simulink model "case1"  (R2024b)
settings: Solver=FixedStepAuto  StartTime=0  StopTime=1  FixedStep=1e-7  RelTol=1e-3
values from neighbouring files (symbols this model uses):
  SG_D_1_D = 0.01056    [IEEE9_case_parameters.m]    (also in case1_parameters.m; case2_parameters.m; case3_parameters.m; case4_parameters.m)
  SG_D_1_EnableSaturation = 0    [IEEE9_case_parameters.m]    (also in case1_parameters.m; case2_parameters.m; case3_parameters.m; case4_parameters.m)
  SG_D_1_f0 = 60    [IEEE9_case_parameters.m]    (also in case1_parameters.m; case2_parameters.m; case3_parameters.m; case4_parameters.m)
  SG_D_1_H = 7.5    [IEEE9_case_parameters.m]    (also in case1_parameters.m; case2_parameters.m; case3_parameters.m; case4_parameters.m)
  SG_D_1_K_A = 20    [IEEE9_case_parameters.m]    (also in case1_parameters.m; case2_parameters.m; case3_parameters.m; case4_parameters.m)
  SG_D_1_K_E = 1.000000e+1    (= 10)    [IEEE9_case_parameters.m]    (also in case1_parameters.m; case2_parameters.m; case3_parameters.m; case4_parameters.m)
  SG_D_1_K_F = 2.363    [IEEE9_case_parameters.m]    (also in case1_parameters.m; case2_parameters.m; case3_parameters.m; case4_parameters.m)
  SG_D_1_K_s = 0.5    [IEEE9_case_parameters.m]    (also in case1_parameters.m = 5; case2_parameters.m = 5; case3_parameters.m = 5; case4_parameters.m = 5)
  SG_D_1_R_a = 0.001088    [IEEE9_case_parameters.m]    (also in case1_parameters.m; case2_parameters.m; case3_parameters.m; case4_parameters.m)
  SG_D_1_S_A = 1    [IEEE9_case_parameters.m]    (also in case1_parameters.m; case2_parameters.m; case3_parameters.m; case4_parameters.m)
  SG_D_1_S_B = 0.103    [IEEE9_case_parameters.m]    (also in case1_parameters.m; case2_parameters.m; case3_parameters.m; case4_parameters.m)
  SG_D_1_S_N = 10.659857    [IEEE9_case_parameters.m]    (also in case1_parameters.m; case2_parameters.m; case3_parameters.m; case4_parameters.m)
  SG_D_1_SpeedPara = 200    [IEEE9_case_parameters.m]    (also in case1_parameters.m; case2_parameters.m; case3_parameters.m; case4_parameters.m)
  SG_D_1_T_0 = 0.720173    [IEEE9_case_parameters.m]    (also in case1_parameters.m = 0.755522; case2_parameters.m = 0.808931; case3_parameters.m = 0.869402; case4_parameters.m = 0.729316)
  SG_D_1_T_1 = 0.3    [IEEE9_case_parameters.m]    (also in case1_parameters.m; case2_parameters.m; case3_parameters.m; case4_parameters.m)
  SG_D_1_T_2 = 0.05    [IEEE9_case_parameters.m]    (also in case1_parameters.m; case2_parameters.m; case3_parameters.m; case4_parameters.m)
  SG_D_1_T_3 = 0.02    [IEEE9_case_parameters.m]    (also in case1_parameters.m; case2_parameters.m; case3_parameters.m; case4_parameters.m)
  SG_D_1_T_4 = 0.005    [IEEE9_case_parameters.m]    (also in case1_parameters.m; case2_parameters.m; case3_parameters.m; case4_parameters.m)
  SG_D_1_T_A = 0.02    [IEEE9_case_parameters.m]    (also in case1_parameters.m; case2_parameters.m; case3_parameters.m; case4_parameters.m)
  SG_D_1_T_dd = 8.000000e+0    (= 8)    [IEEE9_case_parameters.m]    (also in case1_parameters.m; case2_parameters.m; case3_parameters.m; case4_parameters.m)
  SG_D_1_T_ddd = 0.04    [IEEE9_case_parameters.m]    (also in case1_parameters.m; case2_parameters.m; case3_parameters.m; case4_parameters.m)
  SG_D_1_T_E = 0.314    [IEEE9_case_parameters.m]    (also in case1_parameters.m; case2_parameters.m; case3_parameters.m; case4_parameters.m)
  SG_D_1_T_F = 0.35    [IEEE9_case_parameters.m]    (also in case1_parameters.m; case2_parameters.m; case3_parameters.m; case4_parameters.m)
  SG_D_1_T_qd = 0.8    [IEEE9_case_parameters.m]    (also in case1_parameters.m; case2_parameters.m; case3_parameters.m; case4_parameters.m)
  SG_D_1_T_qdd = 0.02    [IEEE9_case_parameters.m]    (also in case1_parameters.m; case2_parameters.m; case3_parameters.m; case4_parameters.m)
  SG_D_1_T_speed = 0.1    [IEEE9_case_parameters.m]    (also in case1_parameters.m = 200; case2_parameters.m = 200; case3_parameters.m = 200; case4_parameters.m = 200)
  SG_D_1_T_w = 0.5    [IEEE9_case_parameters.m]    (also in case1_parameters.m; case2_parameters.m; case3_parameters.m; case4_parameters.m)
  SG_D_1_V_ref = 1.990276    [IEEE9_case_parameters.m]    (also in case1_parameters.m = 2.042296; case2_parameters.m = 2.051388; case3_parameters.m = 2.089584; case4_parameters.m = 2.01845)
  SG_D_1_w_ref = 376.991118    [IEEE9_case_parameters.m]    (also in case1_parameters.m; case2_parameters.m; case3_parameters.m; case4_parameters.m)
  SG_D_1_wb = 6.000000e+1    (= 60)    [IEEE9_case_parameters.m]    (also in case1_parameters.m; case2_parameters.m; case3_parameters.m; case4_parameters.m)
  SG_D_1_x_d = 1.9    [IEEE9_case_parameters.m]    (also in case1_parameters.m; case2_parameters.m; case3_parameters.m; case4_parameters.m)
  SG_D_1_x_dd = 0.302    [IEEE9_case_parameters.m]    (also in case1_parameters.m; case2_parameters.m; case3_parameters.m; case4_parameters.m)
  SG_D_1_x_ddd = 0.204    [IEEE9_case_parameters.m]    (also in case1_parameters.m; case2_parameters.m; case3_parameters.m; case4_parameters.m)
  SG_D_1_x_l = 0.05    [IEEE9_case_parameters.m]    (also in case1_parameters.m; case2_parameters.m; case3_parameters.m; case4_parameters.m)
  SG_D_1_x_q = 1.3    [IEEE9_case_parameters.m]    (also in case1_parameters.m; case2_parameters.m; case3_parameters.m; case4_parameters.m)
  SG_D_1_x_qd = 0.5    [IEEE9_case_parameters.m]    (also in case1_parameters.m; case2_parameters.m; case3_parameters.m; case4_parameters.m)
  SG_D_1_x_qdd = 0.3    [IEEE9_case_parameters.m]    (also in case1_parameters.m; case2_parameters.m; case3_parameters.m; case4_parameters.m)
  SG_D_2_D = 0.02    [IEEE9_case_parameters.m]    (also in case1_parameters.m; case2_parameters.m; case3_parameters.m; case4_parameters.m)
  SG_D_2_EnableSaturation = 0    [IEEE9_case_parameters.m]    (also in case1_parameters.m; case2_parameters.m; case3_parameters.m; case4_parameters.m)
  SG_D_2_f0 = 60    [IEEE9_case_parameters.m]    (also in case1_parameters.m; case2_parameters.m; case3_parameters.m; case4_parameters.m)
  SG_D_2_H = 8.000000e+0    (= 8)    [IEEE9_case_parameters.m]    (also in case1_parameters.m; case2_parameters.m; case3_parameters.m; case4_parameters.m)
  SG_D_2_K_A = 20    [IEEE9_case_parameters.m]    (also in case1_parameters.m; case2_parameters.m; case3_parameters.m; case4_parameters.m)
  SG_D_2_K_E = 1.000000e+1    (= 10)    [IEEE9_case_parameters.m]    (also in case1_parameters.m; case2_parameters.m; case3_parameters.m; case4_parameters.m)
  SG_D_2_K_F = 2.363    [IEEE9_case_parameters.m]    (also in case1_parameters.m; case2_parameters.m; case3_parameters.m; case4_parameters.m)
  SG_D_2_K_s = 0.5    [IEEE9_case_parameters.m]    (also in case1_parameters.m = 4; case2_parameters.m = 4; case3_parameters.m = 4; case4_parameters.m = 4)
  SG_D_2_R_a = 0.001088    [IEEE9_case_parameters.m]    (also in case1_parameters.m; case2_parameters.m; case3_parameters.m; case4_parameters.m)
  SG_D_2_S_A = 1    [IEEE9_case_parameters.m]    (also in case1_parameters.m; case2_parameters.m; case3_parameters.m; case4_parameters.m)
  SG_D_2_S_B = 0.103    [IEEE9_case_parameters.m]    (also in case1_parameters.m; case2_parameters.m; case3_parameters.m; case4_parameters.m)
  SG_D_2_S_N = 10.659857    [IEEE9_case_parameters.m]    (also in case1_parameters.m; case2_parameters.m; case3_parameters.m; case4_parameters.m)
  SG_D_2_SpeedPara = 200    [IEEE9_case_parameters.m]    (also in case1_parameters.m; case2_parameters.m; case3_parameters.m; case4_parameters.m)
  SG_D_2_T_0 = 1.632913    [IEEE9_case_parameters.m]    (also in case1_parameters.m = 1.632925; case2_parameters.m = 1.632915; case3_parameters.m = 1.632914; case4_parameters.m = 1.632927)
  SG_D_2_T_1 = 0.2    [IEEE9_case_parameters.m]    (also in case1_parameters.m; case2_parameters.m; case3_parameters.m; case4_parameters.m)
  SG_D_2_T_2 = 0.05    [IEEE9_case_parameters.m]    (also in case1_parameters.m; case2_parameters.m; case3_parameters.m; case4_parameters.m)
  SG_D_2_T_3 = 0.02    [IEEE9_case_parameters.m]    (also in case1_parameters.m; case2_parameters.m; case3_parameters.m; case4_parameters.m)
  SG_D_2_T_4 = 0.005    [IEEE9_case_parameters.m]    (also in case1_parameters.m; case2_parameters.m; case3_parameters.m; case4_parameters.m)
  SG_D_2_T_A = 0.02    [IEEE9_case_parameters.m]    (also in case1_parameters.m; case2_parameters.m; case3_parameters.m; case4_parameters.m)
  SG_D_2_T_dd = 7.9    [IEEE9_case_parameters.m]    (also in case1_parameters.m; case2_parameters.m; case3_parameters.m; case4_parameters.m)
  SG_D_2_T_ddd = 0.04    [IEEE9_case_parameters.m]    (also in case1_parameters.m; case2_parameters.m; case3_parameters.m; case4_parameters.m)
  SG_D_2_T_E = 0.314    [IEEE9_case_parameters.m]    (also in case1_parameters.m; case2_parameters.m; case3_parameters.m; case4_parameters.m)
  SG_D_2_T_F = 0.35    [IEEE9_case_parameters.m]    (also in case1_parameters.m; case2_parameters.m; case3_parameters.m; case4_parameters.m)
  SG_D_2_T_qd = 0.8    [IEEE9_case_parameters.m]    (also in case1_parameters.m; case2_parameters.m; case3_parameters.m; case4_parameters.m)
  SG_D_2_T_qdd = 0.015    [IEEE9_case_parameters.m]    (also in case1_parameters.m; case2_parameters.m; case3_parameters.m; case4_parameters.m)
  SG_D_2_T_speed = 0.1    [IEEE9_case_parameters.m]    (also in case1_parameters.m = 150; case2_parameters.m = 150; case3_parameters.m = 150; case4_parameters.m = 150)
  SG_D_2_T_w = 0.35    [IEEE9_case_parameters.m]    (also in case1_parameters.m; case2_parameters.m; case3_parameters.m; case4_parameters.m)
  SG_D_2_V_ref = 2.58547    [IEEE9_case_parameters.m]    (also in case1_parameters.m = 2.597896; case2_parameters.m = 2.587136; case3_parameters.m = 2.586042; case4_parameters.m = 2.599679)
  SG_D_2_w_ref = 376.991118    [IEEE9_case_parameters.m]    (also in case1_parameters.m; case2_parameters.m; case3_parameters.m; case4_parameters.m)
  SG_D_2_wb = 6.000000e+1    (= 60)    [IEEE9_case_parameters.m]    (also in case1_parameters.m; case2_parameters.m; case3_parameters.m; case4_parameters.m)
  SG_D_2_x_d = 1.8    [IEEE9_case_parameters.m]    (also in case1_parameters.m; case2_parameters.m; case3_parameters.m; case4_parameters.m)
  SG_D_2_x_dd = 0.302    [IEEE9_case_parameters.m]    (also in case1_parameters.m; case2_parameters.m; case3_parameters.m; case4_parameters.m)
  SG_D_2_x_ddd = 0.204    [IEEE9_case_parameters.m]    (also in case1_parameters.m; case2_parameters.m; case3_parameters.m; case4_parameters.m)
  SG_D_2_x_l = 0.05    [IEEE9_case_parameters.m]    (also in case1_parameters.m; case2_parameters.m; case3_parameters.m; case4_parameters.m)
  SG_D_2_x_q = 1.25    [IEEE9_case_parameters.m]    (also in case1_parameters.m; case2_parameters.m; case3_parameters.m; case4_parameters.m)
  SG_D_2_x_qd = 0.5    [IEEE9_case_parameters.m]    (also in case1_parameters.m; case2_parameters.m; case3_parameters.m; case4_parameters.m)
  SG_D_2_x_qdd = 0.3    [IEEE9_case_parameters.m]    (also in case1_parameters.m; case2_parameters.m; case3_parameters.m; case4_parameters.m)
  SG_D_3_D = 0.02    [IEEE9_case_parameters.m]    (also in case1_parameters.m; case2_parameters.m; case3_parameters.m; case4_parameters.m)
  SG_D_3_EnableSaturation = 0    [IEEE9_case_parameters.m]    (also in case1_parameters.m; case2_parameters.m; case3_parameters.m; case4_parameters.m)
  SG_D_3_f0 = 60    [IEEE9_case_parameters.m]    (also in case1_parameters.m; case2_parameters.m; case3_parameters.m; case4_parameters.m)
  SG_D_3_H = 7.7    [IEEE9_case_parameters.m]    (also in case1_parameters.m; case2_parameters.m; case3_parameters.m; case4_parameters.m)
  SG_D_3_K_A = 20    [IEEE9_case_parameters.m]    (also in case1_parameters.m; case2_parameters.m; case3_parameters.m; case4_parameters.m)
  SG_D_3_K_E = 1.000000e+1    (= 10)    [IEEE9_case_parameters.m]    (also in case1_parameters.m; case2_parameters.m; case3_parameters.m; case4_parameters.m)
  SG_D_3_K_F = 2.363    [IEEE9_case_parameters.m]    (also in case1_parameters.m; case2_parameters.m; case3_parameters.m; case4_parameters.m)
  SG_D_3_K_s = 0.2    [IEEE9_case_parameters.m]    (also in case1_parameters.m = 2; case2_parameters.m = 2; case3_parameters.m = 2; case4_parameters.m = 2)
  SG_D_3_R_a = 0.001088    [IEEE9_case_parameters.m]    (also in case1_parameters.m; case2_parameters.m; case3_parameters.m; case4_parameters.m)
  SG_D_3_S_A = 1    [IEEE9_case_parameters.m]    (also in case1_parameters.m; case2_parameters.m; case3_parameters.m; case4_parameters.m)
  SG_D_3_S_B = 0.103    [IEEE9_case_parameters.m]    (also in case1_parameters.m; case2_parameters.m; case3_parameters.m; case4_parameters.m)
  SG_D_3_S_N = 10.659857    [IEEE9_case_parameters.m]    (also in case1_parameters.m; case2_parameters.m; case3_parameters.m; case4_parameters.m)
  SG_D_3_SpeedPara = 200    [IEEE9_case_parameters.m]    (also in case1_parameters.m; case2_parameters.m; case3_parameters.m; case4_parameters.m)
  SG_D_3_T_0 = 0.850788    [IEEE9_case_parameters.m]    (also in case1_parameters.m = 0.850786; case2_parameters.m = 0.850787; case3_parameters.m; case4_parameters.m = 0.850786)
  SG_D_3_T_1 = 0.2    [IEEE9_case_parameters.m]    (also in case1_parameters.m; case2_parameters.m; case3_parameters.m; case4_parameters.m)
  SG_D_3_T_2 = 0.05    [IEEE9_case_parameters.m]    (also in case1_parameters.m; case2_parameters.m; case3_parameters.m; case4_parameters.m)
  SG_D_3_T_3 = 0.02    [IEEE9_case_parameters.m]    (also in case1_parameters.m; case2_parameters.m; case3_parameters.m; case4_parameters.m)
  SG_D_3_T_4 = 0.005    [IEEE9_case_parameters.m]    (also in case1_parameters.m; case2_parameters.m; case3_parameters.m; case4_parameters.m)
  SG_D_3_T_A = 0.02    [IEEE9_case_parameters.m]    (also in case1_parameters.m; case2_parameters.m; case3_parameters.m; case4_parameters.m)
  SG_D_3_T_dd = 8.1    [IEEE9_case_parameters.m]    (also in case1_parameters.m; case2_parameters.m; case3_parameters.m; case4_parameters.m)
  SG_D_3_T_ddd = 0.04    [IEEE9_case_parameters.m]    (also in case1_parameters.m; case2_parameters.m; case3_parameters.m; case4_parameters.m)
  SG_D_3_T_E = 0.314    [IEEE9_case_parameters.m]    (also in case1_parameters.m; case2_parameters.m; case3_parameters.m; case4_parameters.m)
  SG_D_3_T_F = 0.35    [IEEE9_case_parameters.m]    (also in case1_parameters.m; case2_parameters.m; case3_parameters.m; case4_parameters.m)
  SG_D_3_T_qd = 0.8    [IEEE9_case_parameters.m]    (also in case1_parameters.m; case2_parameters.m; case3_parameters.m; case4_parameters.m)
  SG_D_3_T_qdd = 0.015    [IEEE9_case_parameters.m]    (also in case1_parameters.m; case2_parameters.m; case3_parameters.m; case4_parameters.m)
  SG_D_3_T_speed = 0.1    [IEEE9_case_parameters.m]    (also in case1_parameters.m = 180; case2_parameters.m = 180; case3_parameters.m = 180; case4_parameters.m = 180)
  SG_D_3_T_w = 0.4    [IEEE9_case_parameters.m]    (also in case1_parameters.m; case2_parameters.m; case3_parameters.m; case4_parameters.m)
  SG_D_3_V_ref = 1.892727    [IEEE9_case_parameters.m]    (also in case1_parameters.m = 1.906439; case2_parameters.m = 1.895535; case3_parameters.m = 1.892105; case4_parameters.m = 1.906598)
  SG_D_3_w_ref = 376.991118    [IEEE9_case_parameters.m]    (also in case1_parameters.m; case2_parameters.m; case3_parameters.m; case4_parameters.m)
  SG_D_3_wb = 6.000000e+1    (= 60)    [IEEE9_case_parameters.m]    (also in case1_parameters.m; case2_parameters.m; case3_parameters.m; case4_parameters.m)
  SG_D_3_x_d = 1.85    [IEEE9_case_parameters.m]    (also in case1_parameters.m; case2_parameters.m; case3_parameters.m; case4_parameters.m)
  SG_D_3_x_dd = 0.302    [IEEE9_case_parameters.m]    (also in case1_parameters.m; case2_parameters.m; case3_parameters.m; case4_parameters.m)
  SG_D_3_x_ddd = 0.204    [IEEE9_case_parameters.m]    (also in case1_parameters.m; case2_parameters.m; case3_parameters.m; case4_parameters.m)
  SG_D_3_x_l = 0.05    [IEEE9_case_parameters.m]    (also in case1_parameters.m; case2_parameters.m; case3_parameters.m; case4_parameters.m)
  SG_D_3_x_q = 1.2    [IEEE9_case_parameters.m]    (also in case1_parameters.m; case2_parameters.m; case3_parameters.m; case4_parameters.m)
  SG_D_3_x_qd = 0.5    [IEEE9_case_parameters.m]    (also in case1_parameters.m; case2_parameters.m; case3_parameters.m; case4_parameters.m)
  SG_D_3_x_qdd = 0.3    [IEEE9_case_parameters.m]    (also in case1_parameters.m; case2_parameters.m; case3_parameters.m; case4_parameters.m)
(part 11 of 12)

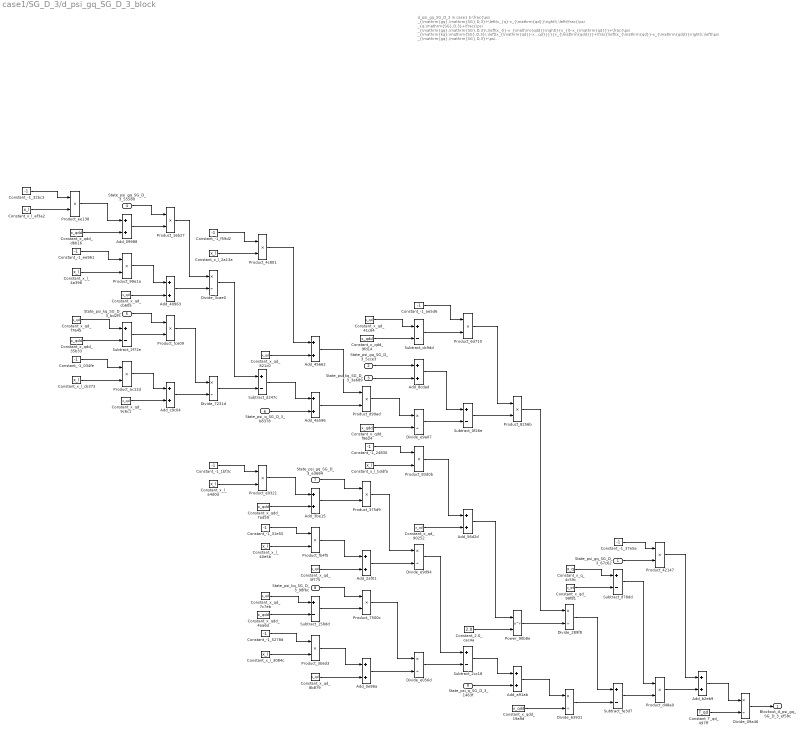
== system case1/SG_D_3/d_psi_gq_SG_D_3_block ==
  note: d_psi_gq_SG_D_3 in case1
      | $-\frac{\psi _{\mathrm{gq},\mathrm{SG},D,3}+\left(x_{q}-x_{\mathrm{qd}}\right)\,\left(\frac{\psi _{q,\mathrm{SG},D,3}+\frac{\psi _{\mathrm{gq},\mathrm{SG},D,3}\,\left(x_{l}-x_{\mathrm{qdd}}\right)}{x_{l}-x_{\mathrm{qd}}}+\frac{\psi _{\mathrm{kq},\mathrm{SG},D,3}\,\left(x_{\mathrm{qd}}-x_{\mathrm{qdd}}\right)}{x_{l}-x_{\mathrm{qd}}}}{x_{\mathrm{qdd}}}+\frac{\left(x_{\mathrm{qd}}-x_{\mathrm{qdd}}\right)\,\left(\psi _{\mathrm{gq},\mathrm{SG},D,3}+\psi _{\mathrm{kq},\mathrm{SG},D,3}+\frac{\left(x_{l}-x_{\mathrm{qd}}\right)\,\left(\psi _{q,\mathrm{SG},D,3}+\frac{\psi _{\mathrm{gq},\mathrm{SG},D,3}\,\left(x_{l}-x_{\mathrm{qdd}}\right)}{x_{l}-x_{\mathrm{qd}}}+\frac{\psi _{\mathrm{kq},\mathrm{SG},D,3}\,\left(x_{\mathrm{qd}}-x_{\mathrm{qdd}}\right)}{x_{l}-x_{\mathrm{qd}}}\right)}{x_{\mathrm{qdd}}}\right)}{{\left(x_{l}-x_{\mathrm{qd}}\right)}^2}\right)}{T_{\mathrm{qd}}}$
      | Automatically generated on 2025-10-31 18:49:40 .
  State_psi_gq_SG_D_3_67c62 : Inport
  State_psi_gq_SG_D_3_5cce3 : Inport  Port=2
  State_psi_kq_SG_D_3_3a689 : Inport  Port=3
  State_psi_gq_SG_D_3_55580 : Inport  Port=4
  State_psi_kq_SG_D_3_bd2f5 : Inport  Port=5
  State_psi_q_SG_D_3_b8378 : Inport  Port=6
  State_psi_gq_SG_D_3_e3684 : Inport  Port=7
  State_psi_kq_SG_D_3_98fbc : Inport  Port=8
  State_psi_q_SG_D_3_1463f : Inport  Port=9
  Add_09988 : Sum
  Add_0e86a : Sum
  Add_2af01 : Sum
  Add_3be15 : Sum
  Add_40963 : Sum
  Add_45662 : Sum
  Add_4a596 : Sum
  Add_56d2d : Sum
  Add_8cdad : Sum
  Add_a91ab : Sum
  Add_b2eb9 : Sum
  Add_c9c04 : Sum
  Constant_-1_034fe : Constant  Value=-1
  Constant_-1_1bf3c : Constant  Value=-1
  Constant_-1_24830 : Constant  Value=-1
  Constant_-1_31e55 : Constant  Value=-1
  Constant_-1_32bc3 : Constant  Value=-1
  Constant_-1_37e5a : Constant  Value=-1
  Constant_-1_5278d : Constant  Value=-1
  Constant_-1_ae5d6 : Constant  Value=-1
  Constant_-1_ee961 : Constant  Value=-1
  Constant_-1_f59d2 : Constant  Value=-1
  Constant_2.0_cac4a : Constant  Value=2.0
  Constant_T_qd_497ff : Constant  Value=T_qd
  Constant_x_l_2a13a : Constant  Value=x_l
  Constant_x_l_3084c : Constant  Value=x_l
  Constant_x_l_40e5b : Constant  Value=x_l
  Constant_x_l_4a396 : Constant  Value=x_l
  Constant_x_l_a4d0d : Constant  Value=x_l
  Constant_x_l_af3a2 : Constant  Value=x_l
  Constant_x_l_b3dfa : Constant  Value=x_l
  Constant_x_l_cb373 : Constant  Value=x_l
  Constant_x_q_4c59c : Constant  Value=x_q
  Constant_x_qd_3f775 : Constant  Value=x_qd
  Constant_x_qd_41c64 : Constant  Value=x_qd
  Constant_x_qd_7c7eb : Constant  Value=x_qd
  Constant_x_qd_821c0 : Constant  Value=x_qd
  Constant_x_qd_8b879 : Constant  Value=x_qd
  Constant_x_qd_90252 : Constant  Value=x_qd
  Constant_x_qd_99f81 : Constant  Value=x_qd
  Constant_x_qd_9c6c1 : Constant  Value=x_qd
  Constant_x_qd_cb605 : Constant  Value=x_qd
  Constant_x_qd_f7645 : Constant  Value=x_qd
  Constant_x_qdd_19a9d : Constant  Value=x_qdd
  Constant_x_qdd_35b33 : Constant  Value=x_qdd
  Constant_x_qdd_4aa6d : Constant  Value=x_qdd
  Constant_x_qdd_7ad59 : Constant  Value=x_qdd
  Constant_x_qdd_9fd14 : Constant  Value=x_qdd
  Constant_x_qdd_dbb16 : Constant  Value=x_qdd
  Constant_x_qdd_f9624 : Constant  Value=x_qdd
  Divide_09a46 : Product  Inputs=*/
  Divide_289f8 : Product  Inputs=*/
  Divide_3cae0 : Product  Inputs=*/
  Divide_63931 : Product  Inputs=*/
  Divide_7231d : Product  Inputs=*/
  Divide_e056d : Product  Inputs=*/
  Divide_e9a07 : Product  Inputs=*/
  Divide_e9d94 : Product  Inputs=*/
  Power_90b8e : Math  Operator=pow
  Product_16b27 : Product
  Product_375d9 : Product
  Product_3b6d3 : Product
  Product_42147 : Product
  Product_4c801 : Product
  Product_6d710 : Product
  Product_7500c : Product
  Product_8256b : Product
  Product_83d0b : Product
  Product_99e1a : Product
  Product_ac12d : Product
  Product_d48a0 : Product
  Product_d99ad : Product
  Product_e0321 : Product
  Product_ee138 : Product
  Product_fb4f5 : Product
  Product_fce09 : Product
  Subtract_0f26e : Sum  Inputs=+-
  Subtract_158dd : Sum  Inputs=+-
  Subtract_2cc18 : Sum  Inputs=+-
  Subtract_2f72e : Sum  Inputs=+-
  Subtract_d247c : Sum  Inputs=+-
  Subtract_d78dd : Sum  Inputs=+-
  Subtract_dc9dd : Sum  Inputs=+-
  Subtract_fe3d7 : Sum  Inputs=+-
  Blockout_d_psi_gq_SG_D_3_ef58c : Outport
  wires:
  Constant_x_l_b3dfa/1 -> Product_83d0b/2
  Constant_x_qd_f7645/1 -> Subtract_2f72e/1
  Add_45662/1 -> Product_d99ad/1
  Constant_-1_32bc3/1 -> Product_ee138/1
  Add_09988/1 -> Product_16b27/2
  Constant_x_qdd_35b33/1 -> Subtract_2f72e/2
  Constant_x_qd_821c0/1 -> Add_45662/2
  Constant_x_l_af3a2/1 -> Product_ee138/2
  Constant_x_l_4a396/1 -> Product_99e1a/2
  Add_0e86a/1 -> Divide_e056d/2
  State_psi_kq_SG_D_3_3a689/1 -> Add_8cdad/2
  Constant_x_qdd_dbb16/1 -> Add_09988/2
  Product_ee138/1 -> Add_09988/1
  Constant_x_qd_8b879/1 -> Add_0e86a/2
  Product_6d710/1 -> Product_8256b/1
  Constant_-1_1bf3c/1 -> Product_e0321/1
  Constant_-1_ee961/1 -> Product_99e1a/1
  Constant_-1_034fe/1 -> Product_ac12d/1
  Constant_x_l_cb373/1 -> Product_ac12d/2
  Constant_-1_ae5d6/1 -> Product_6d710/1
  Constant_-1_37e5a/1 -> Product_42147/1
  State_psi_gq_SG_D_3_55580/1 -> Product_16b27/1
  Product_e0321/1 -> Add_3be15/1
  Product_99e1a/1 -> Add_40963/1
  Product_3b6d3/1 -> Add_0e86a/1
  Constant_x_qd_cb605/1 -> Add_40963/2
  Constant_-1_31e55/1 -> Product_fb4f5/1
  State_psi_kq_SG_D_3_bd2f5/1 -> Product_fce09/1
  Subtract_2f72e/1 -> Product_fce09/2
  Product_ac12d/1 -> Add_c9c04/1
  Add_3be15/1 -> Product_375d9/2
  Add_40963/1 -> Divide_3cae0/2
  Constant_x_qd_9c6c1/1 -> Add_c9c04/2
  Product_16b27/1 -> Divide_3cae0/1
  Constant_T_qd_497ff/1 -> Divide_09a46/2
  Product_fb4f5/1 -> Add_2af01/1
  Product_fce09/1 -> Divide_7231d/1
  Product_7500c/1 -> Divide_e056d/1
  Add_c9c04/1 -> Divide_7231d/2
  Constant_-1_f59d2/1 -> Product_4c801/1
  Constant_x_qdd_f9624/1 -> Divide_e9a07/2
  Constant_x_l_2a13a/1 -> Product_4c801/2
  Divide_3cae0/1 -> Subtract_d247c/1
  Constant_x_qd_99f81/1 -> Subtract_d78dd/2
  Add_2af01/1 -> Divide_e9d94/2
  Divide_7231d/1 -> Subtract_d247c/2
  Constant_x_l_a4d0d/1 -> Product_e0321/2
  Product_4c801/1 -> Add_45662/1
  Constant_-1_24830/1 -> Product_83d0b/1
  Constant_x_l_40e5b/1 -> Product_fb4f5/2
  Subtract_d247c/1 -> Add_4a596/1
  State_psi_q_SG_D_3_b8378/1 -> Add_4a596/2
  Constant_-1_5278d/1 -> Product_3b6d3/1
  Constant_x_qdd_7ad59/1 -> Add_3be15/2
  Constant_x_qd_7c7eb/1 -> Subtract_158dd/1
  Constant_x_qdd_4aa6d/1 -> Subtract_158dd/2
  Constant_x_l_3084c/1 -> Product_3b6d3/2
  Add_4a596/1 -> Product_d99ad/2
  Constant_x_qdd_9fd14/1 -> Subtract_dc9dd/2
  State_psi_gq_SG_D_3_e3684/1 -> Product_375d9/1
  Constant_x_qd_3f775/1 -> Add_2af01/2
  Divide_289f8/1 -> Subtract_fe3d7/1
  State_psi_kq_SG_D_3_98fbc/1 -> Product_7500c/1
  Subtract_158dd/1 -> Product_7500c/2
  Constant_x_qd_41c64/1 -> Subtract_dc9dd/1
  State_psi_gq_SG_D_3_5cce3/1 -> Add_8cdad/1
  Product_d99ad/1 -> Divide_e9a07/1
  Product_375d9/1 -> Divide_e9d94/1
  Subtract_dc9dd/1 -> Product_6d710/2
  Add_8cdad/1 -> Subtract_0f26e/1
  Divide_e9a07/1 -> Subtract_0f26e/2
  Product_83d0b/1 -> Add_56d2d/1
  Constant_x_qd_90252/1 -> Add_56d2d/2
  Divide_e9d94/1 -> Subtract_2cc18/1
  Divide_e056d/1 -> Subtract_2cc18/2
  Subtract_0f26e/1 -> Product_8256b/2
  Add_56d2d/1 -> Power_90b8e/1
  Constant_2.0_cac4a/1 -> Power_90b8e/2
  Subtract_2cc18/1 -> Add_a91ab/1
  State_psi_q_SG_D_3_1463f/1 -> Add_a91ab/2
  Product_8256b/1 -> Divide_289f8/1
  Power_90b8e/1 -> Divide_289f8/2
  Add_a91ab/1 -> Divide_63931/1
  Constant_x_qdd_19a9d/1 -> Divide_63931/2
  Constant_x_q_4c59c/1 -> Subtract_d78dd/1
  Divide_63931/1 -> Subtract_fe3d7/2
  State_psi_gq_SG_D_3_67c62/1 -> Product_42147/2
  Subtract_d78dd/1 -> Product_d48a0/1
  Subtract_fe3d7/1 -> Product_d48a0/2
  Product_42147/1 -> Add_b2eb9/1
  Product_d48a0/1 -> Add_b2eb9/2
  Add_b2eb9/1 -> Divide_09a46/1
  Divide_09a46/1 -> Blockout_d_psi_gq_SG_D_3_ef58c/1

== system case1/SG_D_3/d_psi_kq_SG_D_3_block ==
  note: d_psi_kq_SG_D_3 in case1
      | $-\frac{\psi _{\mathrm{gq},\mathrm{SG},D,3}+\psi _{\mathrm{kq},\mathrm{SG},D,3}+\frac{\left(x_{l}-x_{\mathrm{qd}}\right)\,\left(\psi _{q,\mathrm{SG},D,3}+\frac{\psi _{\mathrm{gq},\mathrm{SG},D,3}\,\left(x_{l}-x_{\mathrm{qdd}}\right)}{x_{l}-x_{\mathrm{qd}}}+\frac{\psi _{\mathrm{kq},\mathrm{SG},D,3}\,\left(x_{\mathrm{qd}}-x_{\mathrm{qdd}}\right)}{x_{l}-x_{\mathrm{qd}}}\right)}{x_{\mathrm{qdd}}}}{T_{\mathrm{qdd}}}$
      | Automatically generated on 2025-10-31 18:49:43 .
  State_psi_gq_SG_D_3_d2333 : Inport
  State_psi_kq_SG_D_3_6b251 : Inport  Port=2
  State_psi_gq_SG_D_3_852d7 : Inport  Port=3
  State_psi_kq_SG_D_3_8c307 : Inport  Port=4
  State_psi_q_SG_D_3_3b888 : Inport  Port=5
  Add_4bba0 : Sum
  Add_58b4c : Sum
  Add_931fd : Sum
  Add_c4f83 : Sum
  Add_e4726 : Sum
  Add_ee729 : Sum
  Constant_-1_2f69e : Constant  Value=-1
  Constant_-1_44d35 : Constant  Value=-1
  Constant_-1_7b10b : Constant  Value=-1
  Constant_-1_a5749 : Constant  Value=-1
  Constant_-1_c2ef4 : Constant  Value=-1
  Constant_T_qdd_8b7ea : Constant  Value=T_qdd
  Constant_x_l_87358 : Constant  Value=x_l
  Constant_x_l_99aa2 : Constant  Value=x_l
  Constant_x_l_d013b : Constant  Value=x_l
  Constant_x_l_fda08 : Constant  Value=x_l
  Constant_x_qd_5ce38 : Constant  Value=x_qd
  Constant_x_qd_80038 : Constant  Value=x_qd
  Constant_x_qd_86b0b : Constant  Value=x_qd
  Constant_x_qd_a3cb9 : Constant  Value=x_qd
  Constant_x_qdd_1b57a : Constant  Value=x_qdd
  Constant_x_qdd_1e56c : Constant  Value=x_qdd
  Constant_x_qdd_b3d62 : Constant  Value=x_qdd
  Divide_14e25 : Product  Inputs=*/
  Divide_2ff9d : Product  Inputs=*/
  Divide_9901f : Product  Inputs=*/
  Divide_bd8a6 : Product  Inputs=*/
  Product_15a3d : Product
  Product_300be : Product
  Product_62232 : Product
  Product_7e491 : Product
  Product_9ff31 : Product
  Product_a4b5c : Product
  Product_b2cfb : Product
  Product_bbfa0 : Product
  Subtract_3fc00 : Sum  Inputs=+-
  Subtract_66370 : Sum  Inputs=+-
  Subtract_b15d7 : Sum  Inputs=+-
  Blockout_d_psi_kq_SG_D_3_28baf : Outport
  wires:
  State_psi_q_SG_D_3_3b888/1 -> Add_4bba0/2
  Constant_-1_c2ef4/1 -> Product_bbfa0/1
  Constant_-1_a5749/1 -> Product_a4b5c/1
  Constant_-1_2f69e/1 -> Product_62232/1
  Constant_x_l_99aa2/1 -> Product_bbfa0/2
  Constant_x_qdd_b3d62/1 -> Add_c4f83/2
  Product_9ff31/1 -> Add_58b4c/1
  Constant_x_l_87358/1 -> Product_a4b5c/2
  Constant_x_qd_86b0b/1 -> Subtract_66370/1
  Product_a4b5c/1 -> Add_c4f83/1
  Constant_x_l_d013b/1 -> Product_15a3d/2
  Constant_x_qdd_1e56c/1 -> Subtract_66370/2
  Constant_-1_44d35/1 -> Product_9ff31/1
  Constant_x_l_fda08/1 -> Product_9ff31/2
  State_psi_gq_SG_D_3_852d7/1 -> Product_b2cfb/1
  Add_c4f83/1 -> Product_b2cfb/2
  Add_4bba0/1 -> Product_7e491/2
  Product_bbfa0/1 -> Add_e4726/1
  Constant_x_qd_80038/1 -> Add_e4726/2
  State_psi_kq_SG_D_3_8c307/1 -> Product_300be/1
  Subtract_66370/1 -> Product_300be/2
  Add_e4726/1 -> Divide_14e25/2
  Constant_x_qd_5ce38/1 -> Add_58b4c/2
  Product_b2cfb/1 -> Divide_14e25/1
  Product_300be/1 -> Divide_bd8a6/1
  Add_58b4c/1 -> Divide_bd8a6/2
  Constant_-1_7b10b/1 -> Product_15a3d/1
  Divide_14e25/1 -> Subtract_3fc00/1
  Add_931fd/1 -> Divide_2ff9d/1
  Divide_bd8a6/1 -> Subtract_3fc00/2
  Divide_2ff9d/1 -> Blockout_d_psi_kq_SG_D_3_28baf/1
  Product_15a3d/1 -> Add_ee729/1
  Constant_x_qd_a3cb9/1 -> Add_ee729/2
  Subtract_3fc00/1 -> Add_4bba0/1
  State_psi_gq_SG_D_3_d2333/1 -> Product_62232/2
  Add_ee729/1 -> Product_7e491/1
  Constant_T_qdd_8b7ea/1 -> Divide_2ff9d/2
  Product_62232/1 -> Subtract_b15d7/1
  State_psi_kq_SG_D_3_6b251/1 -> Subtract_b15d7/2
  Product_7e491/1 -> Divide_9901f/1
  Constant_x_qdd_1b57a/1 -> Divide_9901f/2
  Subtract_b15d7/1 -> Add_931fd/1
  Divide_9901f/1 -> Add_931fd/2

== system case1/SG_D_3/d_psi_q_SG_D_3_block ==
  note: d_psi_q_SG_D_3 in case1
      | $2\,\pi \,f_{0}\,\left(v_{d,\mathrm{SG},D,3}\,\cos\left(\theta _{\mathrm{SG},D,3}\right)+v_{q,\mathrm{SG},D,3}\,\sin\left(\theta _{\mathrm{SG},D,3}\right)-\frac{R_{a}\,\left(\psi _{q,\mathrm{SG},D,3}+\frac{\psi _{\mathrm{gq},\mathrm{SG},D,3}\,\left(x_{l}-x_{\mathrm{qdd}}\right)}{x_{l}-x_{\mathrm{qd}}}+\frac{\psi _{\mathrm{kq},\mathrm{SG},D,3}\,\left(x_{\mathrm{qd}}-x_{\mathrm{qdd}}\right)}{x_{l}-x_{\mathrm{qd}}}\right)}{x_{\mathrm{qdd}}}-\frac{\psi _{d,\mathrm{SG},D,3}\,w_{\mathrm{SG},D,3}}{2\,f_{0}\,\pi }\right)$
      | Automatically generated on 2025-10-31 18:49:26 .
  State_psi_gq_SG_D_3_b4a4d : Inport
  State_psi_kq_SG_D_3_e7fae : Inport  Port=2
  State_psi_q_SG_D_3_1c339 : Inport  Port=3
  Input_v_d_SG_D_3_3c95f : Inport  Port=4
  State_theta_SG_D_3_b412e : Inport  Port=5
  Input_v_q_SG_D_3_30458 : Inport  Port=6
  State_theta_SG_D_3_6cd7f : Inport  Port=7
  State_psi_d_SG_D_3_39242 : Inport  Port=8
  State_w_SG_D_3_33157 : Inport  Port=9
  Add_0a28a : Sum
  Add_1fb4a : Sum
  Add_8a80d : Sum
  Add_8f6d7 : Sum
  Add_b61a3 : Sum
  Constant_-1_09831 : Constant  Value=-1
  Constant_-1_40f79 : Constant  Value=-1
  Constant_-1_7d572 : Constant  Value=-1
  Constant_-2.0_37784 : Constant  Value=-2.0
  Constant_2.0_33906 : Constant  Value=2.0
  Constant_R_a_c673f : Constant  Value=R_a
  Constant_f0_3483c : Constant  Value=f0
  Constant_f0_e42c1 : Constant  Value=f0
  Constant_pi_25a8b : Constant  Value=pi
  Constant_pi_8fec9 : Constant  Value=pi
  Constant_x_l_6b2fb : Constant  Value=x_l
  Constant_x_l_86c92 : Constant  Value=x_l
  Constant_x_l_e01b2 : Constant  Value=x_l
  Constant_x_qd_01ec4 : Constant  Value=x_qd
  Constant_x_qd_6f222 : Constant  Value=x_qd
  Constant_x_qd_86970 : Constant  Value=x_qd
  Constant_x_qdd_033a0 : Constant  Value=x_qdd
  Constant_x_qdd_43d51 : Constant  Value=x_qdd
  Constant_x_qdd_c6aeb : Constant  Value=x_qdd
  Divide_03a1d : Product  Inputs=*/
  Divide_1b431 : Product  Inputs=*/
  Divide_876d5 : Product  Inputs=*/
  Divide_96f7b : Product  Inputs=*/
  MathFunc_cos_99fba : Trigonometry  Operator=cos
  MathFunc_sin_92f53 : Trigonometry
  Product_1a6b3 : Product
  Product_1b548 : Product
  Product_3a97b : Product
  Product_43277 : Product
  Product_692ab : Product
  Product_6ba89 : Product
  Product_91de5 : Product
  Product_984a4 : Product
  Product_a08c0 : Product
  Product_b7b95 : Product
  Product_b9ec1 : Product
  Product_e2263 : Product
  Product_ef29d : Product
  Product_f3098 : Product
  Subtract_16a69 : Sum  Inputs=+-
  Subtract_19dca : Sum  Inputs=+-
  Subtract_55713 : Sum  Inputs=+-
  Subtract_a9ca8 : Sum  Inputs=+-
  Blockout_d_psi_q_SG_D_3_3a763 : Outport
  wires:
  Constant_x_qd_86970/1 -> Subtract_a9ca8/1
  Constant_pi_8fec9/1 -> Product_f3098/2
  Product_1a6b3/1 -> Divide_96f7b/1
  Constant_x_l_e01b2/1 -> Product_43277/2
  Constant_f0_e42c1/1 -> Product_3a97b/2
  State_w_SG_D_3_33157/1 -> Product_e2263/2
  Constant_-1_7d572/1 -> Product_984a4/1
  Constant_x_qdd_033a0/1 -> Add_0a28a/2
  Input_v_d_SG_D_3_3c95f/1 -> Product_6ba89/1
  Constant_x_qdd_c6aeb/1 -> Subtract_a9ca8/2
  Constant_x_l_86c92/1 -> Product_984a4/2
  Divide_1b431/1 -> Add_8f6d7/2
  Product_984a4/1 -> Add_0a28a/1
  Constant_2.0_33906/1 -> Product_f3098/1
  Add_8a80d/1 -> Product_1a6b3/2
  Constant_-1_40f79/1 -> Product_43277/1
  Constant_x_qd_01ec4/1 -> Add_1fb4a/2
  Constant_-1_09831/1 -> Product_1b548/1
  Subtract_16a69/1 -> Subtract_55713/1
  Constant_x_l_6b2fb/1 -> Product_1b548/2
  Subtract_55713/1 -> Add_8f6d7/1
  Constant_f0_3483c/1 -> Product_b9ec1/2
  State_theta_SG_D_3_6cd7f/1 -> MathFunc_sin_92f53/1
  Constant_x_qd_6f222/1 -> Add_b61a3/2
  State_psi_gq_SG_D_3_b4a4d/1 -> Product_a08c0/1
  Add_0a28a/1 -> Product_a08c0/2
  Product_f3098/1 -> Product_b9ec1/1
  Product_43277/1 -> Add_b61a3/1
  State_psi_kq_SG_D_3_e7fae/1 -> Product_ef29d/1
  Subtract_a9ca8/1 -> Product_ef29d/2
  Product_1b548/1 -> Add_1fb4a/1
  MathFunc_sin_92f53/1 -> Product_692ab/2
  Product_a08c0/1 -> Divide_876d5/1
  Product_b9ec1/1 -> Divide_1b431/2
  Add_b61a3/1 -> Divide_876d5/2
  Product_ef29d/1 -> Divide_03a1d/1
  Add_1fb4a/1 -> Divide_03a1d/2
  Input_v_q_SG_D_3_30458/1 -> Product_692ab/1
  Divide_876d5/1 -> Subtract_19dca/1
  Subtract_19dca/1 -> Add_8a80d/1
  Divide_03a1d/1 -> Subtract_19dca/2
  Divide_96f7b/1 -> Subtract_16a69/1
  State_psi_q_SG_D_3_1c339/1 -> Add_8a80d/2
  Product_692ab/1 -> Subtract_55713/2
  Constant_R_a_c673f/1 -> Product_1a6b3/1
  State_theta_SG_D_3_b412e/1 -> MathFunc_cos_99fba/1
  Constant_x_qdd_43d51/1 -> Divide_96f7b/2
  MathFunc_cos_99fba/1 -> Product_6ba89/2
  Constant_-2.0_37784/1 -> Product_91de5/1
  Product_6ba89/1 -> Subtract_16a69/2
  State_psi_d_SG_D_3_39242/1 -> Product_e2263/1
  Constant_pi_25a8b/1 -> Product_91de5/2
  Product_e2263/1 -> Divide_1b431/1
  Product_91de5/1 -> Product_3a97b/1
  Product_3a97b/1 -> Product_b7b95/1
  Add_8f6d7/1 -> Product_b7b95/2
  Product_b7b95/1 -> Blockout_d_psi_q_SG_D_3_3a763/1

== system case1/SG_D_3/d_theta_SG_D_3_block ==
  note: d_theta_SG_D_3 in case1
      | $w_{\mathrm{SG},D,3}-2\,\pi \,f_{0}$
      | Automatically generated on 2025-10-31 18:49:51 .
  State_w_SG_D_3_f4ecf : Inport
  Add_96a9b : Sum
  Constant_-2.0_896de : Constant  Value=-2.0
  Constant_f0_472a7 : Constant  Value=f0
  Constant_pi_f7a3a : Constant  Value=pi
  Product_17f2b : Product
  Product_afb3b : Product
  Blockout_d_theta_SG_D_3_d61c2 : Outport
  wires:
  Constant_-2.0_896de/1 -> Product_17f2b/1
  Constant_pi_f7a3a/1 -> Product_17f2b/2
  State_w_SG_D_3_f4ecf/1 -> Add_96a9b/2
  Product_17f2b/1 -> Product_afb3b/1
  Constant_f0_472a7/1 -> Product_afb3b/2
  Product_afb3b/1 -> Add_96a9b/1
  Add_96a9b/1 -> Blockout_d_theta_SG_D_3_d61c2/1

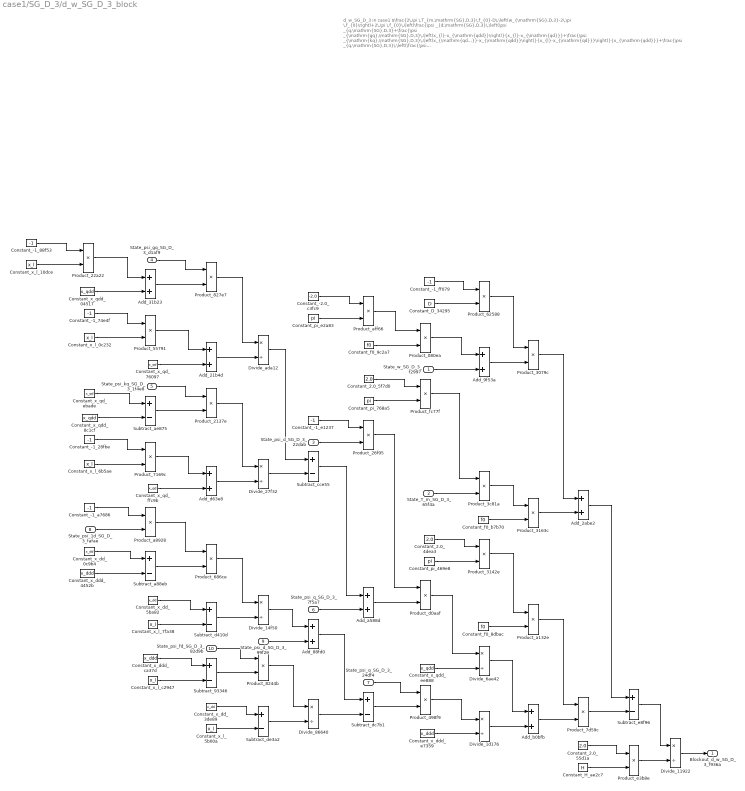
== system case1/SG_D_3/d_w_SG_D_3_block ==
  note: d_w_SG_D_3 in case1
      | $\frac{2\,\pi \,T_{m,\mathrm{SG},D,3}\,f_{0}-D\,\left(w_{\mathrm{SG},D,3}-2\,\pi \,f_{0}\right)+2\,\pi \,f_{0}\,\left(\frac{\psi _{d,\mathrm{SG},D,3}\,\left(\psi _{q,\mathrm{SG},D,3}+\frac{\psi _{\mathrm{gq},\mathrm{SG},D,3}\,\left(x_{l}-x_{\mathrm{qdd}}\right)}{x_{l}-x_{\mathrm{qd}}}+\frac{\psi _{\mathrm{kq},\mathrm{SG},D,3}\,\left(x_{\mathrm{qd}}-x_{\mathrm{qdd}}\right)}{x_{l}-x_{\mathrm{qd}}}\right)}{x_{\mathrm{qdd}}}+\frac{\psi _{q,\mathrm{SG},D,3}\,\left(\frac{\psi _{\mathrm{1d},\mathrm{SG},D,3}\,\left(x_{\mathrm{dd}}-x_{\mathrm{ddd}}\right)}{x_{\mathrm{dd}}-x_{l}}-\psi _{d,\mathrm{SG},D,3}+\frac{\psi _{\mathrm{fd},\mathrm{SG},D,3}\,\left(x_{\mathrm{ddd}}-x_{l}\right)}{x_{\mathrm{dd}}-x_{l}}\right)}{x_{\mathrm{ddd}}}\right)}{2\,H}$
      | Automatically generated on 2025-10-31 18:49:50 .
  State_w_SG_D_3_f2997 : Inport
  State_T_m_SG_D_3_65f4a : Inport  Port=2
  State_psi_d_SG_D_3_22dab : Inport  Port=3
  State_psi_gq_SG_D_3_d1af9 : Inport  Port=4
  State_psi_kq_SG_D_3_1f4e8 : Inport  Port=5
  State_psi_q_SG_D_3_7f5a7 : Inport  Port=6
  State_psi_q_SG_D_3_24df4 : Inport  Port=7
  State_psi_1d_SG_D_3_fafae : Inport  Port=8
  State_psi_d_SG_D_3_99f2e : Inport  Port=9
  State_psi_fd_SG_D_3_82d9b : Inport  Port=10
  Add_21b4d : Sum
  Add_2abe2 : Sum
  Add_31b23 : Sum
  Add_88fd0 : Sum
  Add_9f53a : Sum
  Add_a588d : Sum
  Add_b0bfb : Sum
  Add_d63e8 : Sum
  Constant_-1_28fbe : Constant  Value=-1
  Constant_-1_74e4f : Constant  Value=-1
  Constant_-1_88f53 : Constant  Value=-1
  Constant_-1_a7686 : Constant  Value=-1
  Constant_-1_e1237 : Constant  Value=-1
  Constant_-1_ff079 : Constant  Value=-1
  Constant_-2.0_c3fc9 : Constant  Value=-2.0
  Constant_2.0_4dea3 : Constant  Value=2.0
  Constant_2.0_55d1a : Constant  Value=2.0
  Constant_2.0_5f7d0 : Constant  Value=2.0
  Constant_D_34295 : Constant  Value=D
  Constant_H_ae2c7 : Constant  Value=H
  Constant_f0_8dbac : Constant  Value=f0
  Constant_f0_9c2a7 : Constant  Value=f0
  Constant_f0_b7b70 : Constant  Value=f0
  Constant_pi_469e8 : Constant  Value=pi
  Constant_pi_768a5 : Constant  Value=pi
  Constant_pi_e2a83 : Constant  Value=pi
  Constant_x_dd_0c9b4 : Constant  Value=x_dd
  Constant_x_dd_3de89 : Constant  Value=x_dd
  Constant_x_dd_5ba82 : Constant  Value=x_dd
  Constant_x_ddd_4452b : Constant  Value=x_ddd
  Constant_x_ddd_ca37d : Constant  Value=x_ddd
  Constant_x_ddd_e7359 : Constant  Value=x_ddd
  Constant_x_l_0c232 : Constant  Value=x_l
  Constant_x_l_10dce : Constant  Value=x_l
  Constant_x_l_5b00a : Constant  Value=x_l
  Constant_x_l_6b5ae : Constant  Value=x_l
  Constant_x_l_7fa38 : Constant  Value=x_l
  Constant_x_l_c2947 : Constant  Value=x_l
  Constant_x_qd_76097 : Constant  Value=x_qd
  Constant_x_qd_ebade : Constant  Value=x_qd
  Constant_x_qd_ffc9b : Constant  Value=x_qd
  Constant_x_qdd_04517 : Constant  Value=x_qdd
  Constant_x_qdd_8c1cf : Constant  Value=x_qdd
  Constant_x_qdd_ee888 : Constant  Value=x_qdd
  Divide_11922 : Product  Inputs=*/
  Divide_14f50 : Product  Inputs=*/
  Divide_1d176 : Product  Inputs=*/
  Divide_27f32 : Product  Inputs=*/
  Divide_6ae42 : Product  Inputs=*/
  Divide_86640 : Product  Inputs=*/
  Divide_ada12 : Product  Inputs=*/
  Product_080ea : Product
  Product_2137e : Product
  Product_22a22 : Product
  Product_26f95 : Product
  Product_3079c : Product
  Product_3142e : Product
  Product_3163c : Product
  Product_3c81a : Product
  Product_498f9 : Product
  Product_55791 : Product
  Product_62588 : Product
  Product_686ce : Product
  Product_7169c : Product
  Product_7d59c : Product
  Product_8244b : Product
  Product_827e7 : Product
  Product_a132e : Product
  Product_a8928 : Product
  Product_aff66 : Product
  Product_d0aaf : Product
  Product_e3b8e : Product
  Product_fc77f : Product
  Subtract_93346 : Sum  Inputs=+-
  Subtract_a88eb : Sum  Inputs=+-
  Subtract_ae875 : Sum  Inputs=+-
  Subtract_cce55 : Sum  Inputs=+-
  Subtract_d410d : Sum  Inputs=+-
  Subtract_dc7b1 : Sum  Inputs=+-
  Subtract_de3a2 : Sum  Inputs=+-
  Subtract_e8f96 : Sum  Inputs=+-
  Blockout_d_w_SG_D_3_f936a : Outport
  wires:
  Constant_x_qd_ebade/1 -> Subtract_ae875/1
  Subtract_a88eb/1 -> Product_686ce/2
  Subtract_e8f96/1 -> Divide_11922/1
  Constant_-1_88f53/1 -> Product_22a22/1
  Add_31b23/1 -> Product_827e7/2
  Constant_x_qdd_8c1cf/1 -> Subtract_ae875/2
  Subtract_93346/1 -> Product_8244b/2
  Constant_x_l_10dce/1 -> Product_22a22/2
  State_psi_d_SG_D_3_99f2e/1 -> Add_88fd0/2
  Add_21b4d/1 -> Divide_ada12/2
  Constant_x_dd_5ba82/1 -> Subtract_d410d/1
  Constant_x_l_0c232/1 -> Product_55791/2
  Constant_-1_ff079/1 -> Product_62588/1
  Divide_86640/1 -> Subtract_dc7b1/2
  Constant_x_ddd_4452b/1 -> Subtract_a88eb/2
  Constant_x_qdd_04517/1 -> Add_31b23/2
  Constant_pi_768a5/1 -> Product_fc77f/2
  Product_22a22/1 -> Add_31b23/1
  Constant_-2.0_c3fc9/1 -> Product_aff66/1
  Constant_-1_74e4f/1 -> Product_55791/1
  Constant_2.0_4dea3/1 -> Product_3142e/1
  Product_aff66/1 -> Product_080ea/1
  Constant_-1_28fbe/1 -> Product_7169c/1
  Subtract_cce55/1 -> Add_a588d/1
  Constant_x_l_6b5ae/1 -> Product_7169c/2
  Constant_x_l_c2947/1 -> Subtract_93346/2
  Constant_-1_a7686/1 -> Product_a8928/1
  State_psi_1d_SG_D_3_fafae/1 -> Product_a8928/2
  Constant_x_dd_0c9b4/1 -> Subtract_a88eb/1
  Product_a8928/1 -> Product_686ce/1
  State_psi_gq_SG_D_3_d1af9/1 -> Product_827e7/1
  Constant_x_qd_76097/1 -> Add_21b4d/2
  Product_55791/1 -> Add_21b4d/1
  State_psi_kq_SG_D_3_1f4e8/1 -> Product_2137e/1
  Subtract_ae875/1 -> Product_2137e/2
  Product_3142e/1 -> Product_a132e/1
  Product_080ea/1 -> Add_9f53a/1
  Product_7169c/1 -> Add_d63e8/1
  State_psi_q_SG_D_3_24df4/1 -> Product_498f9/1
  Constant_x_qd_ffc9b/1 -> Add_d63e8/2
  Constant_x_l_7fa38/1 -> Subtract_d410d/2
  Constant_x_ddd_ca37d/1 -> Subtract_93346/1
  Constant_x_l_5b00a/1 -> Subtract_de3a2/2
  Product_827e7/1 -> Divide_ada12/1
  Product_2137e/1 -> Divide_27f32/1
  Add_d63e8/1 -> Divide_27f32/2
  Product_686ce/1 -> Divide_14f50/1
  Subtract_d410d/1 -> Divide_14f50/2
  Constant_2.0_5f7d0/1 -> Product_fc77f/1
  State_psi_fd_SG_D_3_82d9b/1 -> Product_8244b/1
  Constant_x_dd_3de89/1 -> Subtract_de3a2/1
  Divide_ada12/1 -> Subtract_cce55/1
  Product_8244b/1 -> Divide_86640/1
  Divide_27f32/1 -> Subtract_cce55/2
  Divide_14f50/1 -> Add_88fd0/1
  Product_7d59c/1 -> Subtract_e8f96/2
  Subtract_de3a2/1 -> Divide_86640/2
  Constant_pi_e2a83/1 -> Product_aff66/2
  Constant_pi_469e8/1 -> Product_3142e/2
  Constant_-1_e1237/1 -> Product_26f95/1
  State_psi_d_SG_D_3_22dab/1 -> Product_26f95/2
  State_psi_q_SG_D_3_7f5a7/1 -> Add_a588d/2
  Add_88fd0/1 -> Subtract_dc7b1/1
  Constant_f0_9c2a7/1 -> Product_080ea/2
  Product_26f95/1 -> Product_d0aaf/1
  Add_a588d/1 -> Product_d0aaf/2
  Subtract_dc7b1/1 -> Product_498f9/2
  Constant_D_34295/1 -> Product_62588/2
  State_w_SG_D_3_f2997/1 -> Add_9f53a/2
  Product_fc77f/1 -> Product_3c81a/1
  State_T_m_SG_D_3_65f4a/1 -> Product_3c81a/2
  Product_d0aaf/1 -> Divide_6ae42/1
  Constant_x_qdd_ee888/1 -> Divide_6ae42/2
  Product_498f9/1 -> Divide_1d176/1
  Constant_x_ddd_e7359/1 -> Divide_1d176/2
  Product_62588/1 -> Product_3079c/1
  Add_9f53a/1 -> Product_3079c/2
  Product_3c81a/1 -> Product_3163c/1
  Constant_f0_b7b70/1 -> Product_3163c/2
  Constant_f0_8dbac/1 -> Product_a132e/2
  Divide_6ae42/1 -> Add_b0bfb/1
  Divide_1d176/1 -> Add_b0bfb/2
  Product_3079c/1 -> Add_2abe2/1
  Product_3163c/1 -> Add_2abe2/2
  Product_a132e/1 -> Product_7d59c/1
  Add_b0bfb/1 -> Product_7d59c/2
  Add_2abe2/1 -> Subtract_e8f96/1
  Constant_2.0_55d1a/1 -> Product_e3b8e/1
  Constant_H_ae2c7/1 -> Product_e3b8e/2
  Product_e3b8e/1 -> Divide_11922/2
  Divide_11922/1 -> Blockout_d_w_SG_D_3_f936a/1

== system case1/SG_D_3/i_d_SG_D_3_block ==
  note: i_d_SG_D_3 in case1
      | $\frac{\sin\left(\theta _{\mathrm{SG},D,3}\right)\,\left(\frac{\psi _{\mathrm{1d},\mathrm{SG},D,3}\,\left(x_{\mathrm{dd}}-x_{\mathrm{ddd}}\right)}{x_{\mathrm{dd}}-x_{l}}-\psi _{d,\mathrm{SG},D,3}+\frac{\psi _{\mathrm{fd},\mathrm{SG},D,3}\,\left(x_{\mathrm{ddd}}-x_{l}\right)}{x_{\mathrm{dd}}-x_{l}}\right)}{x_{\mathrm{ddd}}}-\frac{\cos\left(\theta _{\mathrm{SG},D,3}\right)\,\left(\psi _{q,\mathrm{SG},D,3}+\frac{\psi _{\mathrm{gq},\mathrm{SG},D,3}\,\left(x_{l}-x_{\mathrm{qdd}}\right)}{x_{l}-x_{\mathrm{qd}}}+\frac{\psi _{\mathrm{kq},\mathrm{SG},D,3}\,\left(x_{\mathrm{qd}}-x_{\mathrm{qdd}}\right)}{x_{l}-x_{\mathrm{qd}}}\right)}{x_{\mathrm{qdd}}}$
      | Automatically generated on 2025-10-31 18:50:01 .
  State_psi_gq_SG_D_3_aa812 : Inport
  State_psi_kq_SG_D_3_86816 : Inport  Port=2
  State_psi_q_SG_D_3_bb946 : Inport  Port=3
  State_theta_SG_D_3_b0af7 : Inport  Port=4
  State_psi_1d_SG_D_3_8f98b : Inport  Port=5
  State_psi_d_SG_D_3_8ce12 : Inport  Port=6
  State_psi_fd_SG_D_3_34c08 : Inport  Port=7
  State_theta_SG_D_3_03ed0 : Inport  Port=8
  Add_1a7f5 : Sum
  Add_62bb1 : Sum
  Add_65dc5 : Sum
  Add_950ce : Sum
  Add_e3aff : Sum
  Constant_-1_5bb76 : Constant  Value=-1
  Constant_-1_68f6e : Constant  Value=-1
  Constant_-1_6adc0 : Constant  Value=-1
  Constant_-1_db605 : Constant  Value=-1
  Constant_-1_df489 : Constant  Value=-1
  Constant_x_dd_70af2 : Constant  Value=x_dd
  Constant_x_dd_cad32 : Constant  Value=x_dd
  Constant_x_dd_fa01b : Constant  Value=x_dd
  Constant_x_ddd_b3604 : Constant  Value=x_ddd
  Constant_x_ddd_c0bd3 : Constant  Value=x_ddd
  Constant_x_ddd_f5967 : Constant  Value=x_ddd
  Constant_x_l_0b61e : Constant  Value=x_l
  Constant_x_l_0f973 : Constant  Value=x_l
  Constant_x_l_7cebe : Constant  Value=x_l
  Constant_x_l_90582 : Constant  Value=x_l
  Constant_x_l_a1a52 : Constant  Value=x_l
  Constant_x_l_d6293 : Constant  Value=x_l
  Constant_x_qd_0c097 : Constant  Value=x_qd
  Constant_x_qd_e7182 : Constant  Value=x_qd
  Constant_x_qd_f4d67 : Constant  Value=x_qd
  Constant_x_qdd_0ad4a : Constant  Value=x_qdd
  Constant_x_qdd_b0096 : Constant  Value=x_qdd
  Constant_x_qdd_cf8b0 : Constant  Value=x_qdd
  Divide_0bbfa : Product  Inputs=*/
  Divide_2585d : Product  Inputs=*/
  Divide_3721a : Product  Inputs=*/
  Divide_53fc0 : Product  Inputs=*/
  Divide_d570a : Product  Inputs=*/
  Divide_e4541 : Product  Inputs=*/
  MathFunc_cos_1a161 : Trigonometry  Operator=cos
  MathFunc_sin_be1c1 : Trigonometry
  Product_0db49 : Product
  Product_20d40 : Product
  Product_5179e : Product
  Product_934b2 : Product
  Product_95a8a : Product
  Product_99415 : Product
  Product_b1572 : Product
  Product_c4ef7 : Product
  Product_cd2bd : Product
  Product_e0d9a : Product
  Product_e3f4a : Product
  Subtract_1e00d : Sum  Inputs=+-
  Subtract_20262 : Sum  Inputs=+-
  Subtract_38401 : Sum  Inputs=+-
  Subtract_57690 : Sum  Inputs=+-
  Subtract_61aab : Sum  Inputs=+-
  Subtract_b45fc : Sum  Inputs=+-
  Subtract_c1b0a : Sum  Inputs=+-
  Subtract_efc40 : Sum  Inputs=+-
  Blockout_i_d_SG_D_3_90043 : Outport
  wires:
  Constant_x_qd_0c097/1 -> Subtract_20262/1
  Subtract_c1b0a/1 -> Blockout_i_d_SG_D_3_90043/1
  Constant_-1_5bb76/1 -> Product_e0d9a/1
  Constant_x_l_0b61e/1 -> Product_b1572/2
  Constant_x_qdd_cf8b0/1 -> Add_950ce/2
  Constant_x_qdd_b0096/1 -> Subtract_20262/2
  Constant_x_l_d6293/1 -> Product_e0d9a/2
  Divide_e4541/1 -> Subtract_c1b0a/1
  Product_e0d9a/1 -> Add_950ce/1
  Constant_x_ddd_c0bd3/1 -> Subtract_57690/2
  Constant_-1_db605/1 -> Product_b1572/1
  Constant_-1_6adc0/1 -> Product_5179e/1
  Constant_x_l_0f973/1 -> Product_5179e/2
  State_psi_1d_SG_D_3_8f98b/1 -> Product_99415/2
  State_psi_gq_SG_D_3_aa812/1 -> Product_0db49/1
  Product_99415/1 -> Product_934b2/1
  Add_950ce/1 -> Product_0db49/2
  Product_b1572/1 -> Add_62bb1/1
  Constant_x_qd_f4d67/1 -> Add_62bb1/2
  State_psi_kq_SG_D_3_86816/1 -> Product_e3f4a/1
  Subtract_61aab/1 -> Divide_0bbfa/2
  Subtract_20262/1 -> Product_e3f4a/2
  Product_5179e/1 -> Add_e3aff/1
  Constant_x_ddd_b3604/1 -> Subtract_1e00d/1
  Constant_x_qd_e7182/1 -> Add_e3aff/2
  Constant_-1_68f6e/1 -> Product_99415/1
  Constant_x_dd_fa01b/1 -> Subtract_57690/1
  Product_0db49/1 -> Divide_53fc0/1
  Add_62bb1/1 -> Divide_53fc0/2
  Product_e3f4a/1 -> Divide_3721a/1
  Add_e3aff/1 -> Divide_3721a/2
  Divide_0bbfa/1 -> Subtract_38401/2
  Subtract_57690/1 -> Product_934b2/2
  State_theta_SG_D_3_b0af7/1 -> MathFunc_cos_1a161/1
  Constant_x_dd_cad32/1 -> Subtract_efc40/1
  Product_20d40/1 -> Product_cd2bd/1
  Constant_x_l_7cebe/1 -> Subtract_efc40/2
  Add_65dc5/1 -> Subtract_38401/1
  Constant_x_l_90582/1 -> Subtract_1e00d/2
  State_theta_SG_D_3_03ed0/1 -> MathFunc_sin_be1c1/1
  Divide_53fc0/1 -> Subtract_b45fc/1
  Add_1a7f5/1 -> Product_20d40/2
  Divide_3721a/1 -> Subtract_b45fc/2
  Product_934b2/1 -> Divide_d570a/1
  Subtract_efc40/1 -> Divide_d570a/2
  State_psi_fd_SG_D_3_34c08/1 -> Product_c4ef7/1
  Divide_2585d/1 -> Subtract_c1b0a/2
  Subtract_1e00d/1 -> Product_c4ef7/2
  Constant_x_dd_70af2/1 -> Subtract_61aab/1
  Subtract_b45fc/1 -> Add_1a7f5/1
  Constant_x_l_a1a52/1 -> Subtract_61aab/2
  Constant_-1_df489/1 -> Product_20d40/1
  State_psi_q_SG_D_3_bb946/1 -> Add_1a7f5/2
  Divide_d570a/1 -> Add_65dc5/1
  State_psi_d_SG_D_3_8ce12/1 -> Add_65dc5/2
  Product_c4ef7/1 -> Divide_0bbfa/1
  MathFunc_cos_1a161/1 -> Product_cd2bd/2
  MathFunc_sin_be1c1/1 -> Product_95a8a/2
  Subtract_38401/1 -> Product_95a8a/1
  Product_cd2bd/1 -> Divide_e4541/1
  Constant_x_qdd_0ad4a/1 -> Divide_e4541/2
  Product_95a8a/1 -> Divide_2585d/1
  Constant_x_ddd_f5967/1 -> Divide_2585d/2
